simulink library "bluetoothLibrary"  (R2015b)
settings: Solver=VariableStepAuto  StartTime=0.0  StopTime=10.0  RelTol=1e-3
settings Model: Creator=dc315  LastModifiedBy=dc315

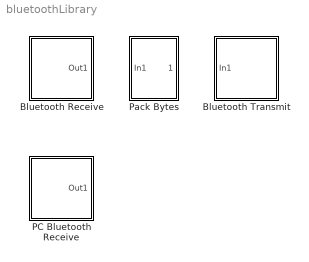
== system bluetoothLibrary ==
  Bluetooth Receive : Subsystem
      mask Display:
      | pic = imread('bluetooth_icon2.jpg');
      | image(pic);
  Bluetooth Transmit : Subsystem  mask{baudRate=9600}
      mask prompts: baudRate "the baud rate, in bits/s:"
      mask TypeOptions baudRate: MATLAB System/baudRate
      mask Display:
      | pic = imread('bluetooth_icon2.jpg');
      | image(pic);
  PC Bluetooth Receive : Subsystem
      mask Display:
      | pic = imread('bluetooth_icon2.jpg');
      | image(pic);
  Pack Bytes : Subsystem  mask{Value=77554433}
      mask prompts: Value "Header"
      mask TypeOptions Value: Constant/Value
      mask Display:
      | pic = imread('pack_icon.jpg');
      | image(pic,'center');

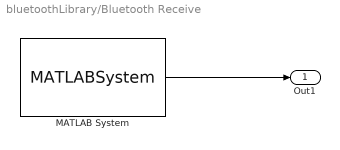
== system bluetoothLibrary/Bluetooth Receive ==
  MATLAB System : MATLABSystem  System=freedomboard.bluetoothIn  baudRate=9600  SimulateUsing=Code generation
      mask Type: freedomboard.bluetoothIn
      mask Display:
      | disp('bluetoothIn');
      | port_label('output',1,'data');
  Out1 : Outport
  wires:
  MATLAB System/1 -> Out1/1

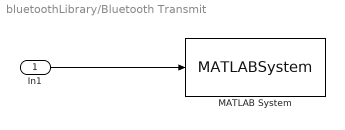
== system bluetoothLibrary/Bluetooth Transmit ==
  In1 : Inport
  MATLAB System : MATLABSystem  System=freedomboard.bluetoothOut  baudRate=baudRate  SimulateUsing=Code generation
      mask Type: freedomboard.bluetoothOut
      mask Display:
      | disp('bluetoothOut');
      | port_label('input',1,'data');
  wires:
  In1/1 -> MATLAB System/1

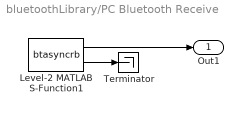
== system bluetoothLibrary/PC Bluetooth Receive ==
  Level-2 MATLAB S-Function1 : M-S-Function  FunctionName=btasyncrb  Parameters='','','','','',[5 1],'double','off','Output last received value',0,0.01
  Terminator : Terminator
  Out1 : Outport
  wires:
  Level-2 MATLAB S-Function1/2 -> Terminator/1
  Level-2 MATLAB S-Function1/1 -> Out1/1

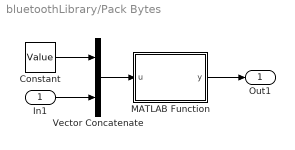
== system bluetoothLibrary/Pack Bytes ==
  In1 : Inport
  Constant : Constant  Value=Value
  MATLAB Function : MATLAB Function  TreatAsAtomicUnit=on
  Vector Concatenate : Concatenate
  Out1 : Outport
  wires:
  In1/1 -> Vector Concatenate/2
  MATLAB Function/1(y) -> Out1/1
  Constant/1 -> Vector Concatenate/1
  Vector Concatenate/1 -> MATLAB Function/1(u)

== matlab function bluetoothLibrary/Pack Bytes/MATLAB Function ==
  data: u input; y output
function y = fcn(u)
%#codegen

y = typecast(u,'uint8');
